simulink model "sum_tut1"  (Simulink 4.00)
settings: Solver=FixedStepDiscrete  SolverMode=SingleTasking  StartTime=0.0  StopTime=10.0  RelTol=1e-3
libraries: dspsrcs3 x2
settings Model: LastModifiedBy=dfass  LimitDataPoints=off  ExtModeTrigMode=oneshot  ExtModeArmWhenConnect=off  BlockReductionOpt=off

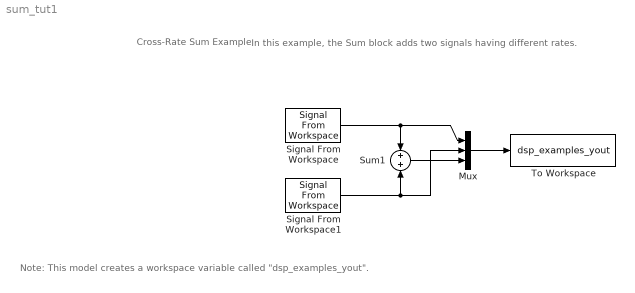
== system sum_tut1 ==
  note: Cross-Rate Sum Example
  note: In this example, the Sum block adds two signals having
      | different rates.
  note: Note: This model creates a workspace variable called "dsp_examples_yout".
  Mux : Mux  Inputs=3
  Signal From Workspace : dspsrcs3/Signal From Workspace  X=1:10  Ts=1  nsamps=1  OutputAfterFinalValue=Setting To Zero
  Signal From Workspace1 : dspsrcs3/Signal From Workspace  X=1:10  Ts=2  nsamps=1  OutputAfterFinalValue=Setting To Zero
  Sum1 : Sum  Inputs=++  SaturateOnIntegerOverflow=on
  To Workspace : ToWorkspace  VariableName=dsp_examples_yout  SampleTime=-1  SaveFormat=Array
  wires:
  Sum1/1 -> Mux/3
  Signal From Workspace/1 -> Sum1/1, Mux/1
  Signal From Workspace1/1 -> Sum1/2, Mux/2
  Mux/1 -> To Workspace/1
